simulink model "my_DC_motor_model"  (R2022b)
settings: Solver=FixedStepAuto  StartTime=0.0  StopTime=5  FixedStep=0.0001  RelTol=1e-3
values from neighbouring files (symbols this model uses):
  B_motor = 1.9099e-4    (= 0.00019099)    [DC_motor_init.m]    (also in LOAD_ROBOT_DATA.m = 0.000678; circular_interp.m = 0.000678; computed_torque_control.m; create_model_tree.m)
  J_rotor = 2118.45e-7    (= 0.000211845)    [DC_motor_init.m]    (also in LOAD_ROBOT_DATA.m = 0.0125; circular_interp.m = 0.0125; computed_torque_control.m; create_model_tree.m)
  Ke = 0.08    [DC_motor_init.m]    (also in LOAD_ROBOT_DATA.m = 0.957; circular_interp.m = 0.957; computed_torque_control.m; create_model_tree.m)
  Kt = 0.08    [DC_motor_init.m]    (also in LOAD_ROBOT_DATA.m = 0.957; circular_interp.m = 0.957; computed_torque_control.m; create_model_tree.m)
  L = 0.90e-3    (= 0.0009)    [DC_motor_init.m]    (also in LOAD_ROBOT_DATA.m = 0.0054; circular_interp.m = 0.0054; computed_torque_control.m; create_model_tree.m)
  R = 0.43    [DC_motor_init.m]    (also in LOAD_ROBOT_DATA.m = 1.45; circular_interp.m = 1.45; computed_torque_control.m; create_model_tree.m)
settings Model: Creator=doann  LastModifiedBy=doann

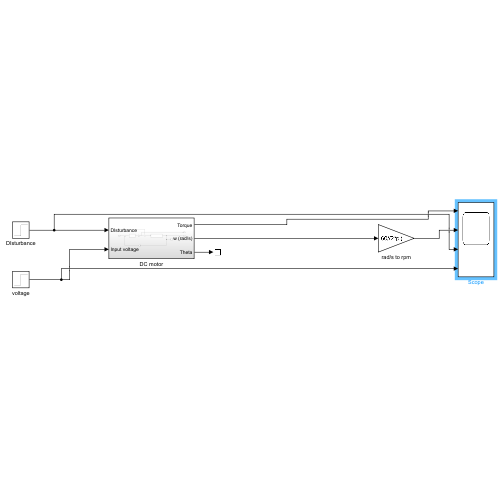
[thumbnail: Simulink's stored preview of the top-level diagram]
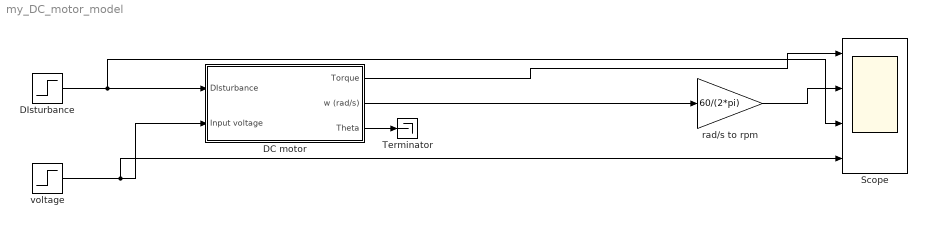
== system my_DC_motor_model ==
  DC motor : Subsystem
  DIsturbance : Step  Time=2.5  After=5  SampleTime=0
  Scope : Scope  NumInputPorts=4
  Terminator : Terminator
  rad/s to rpm : Gain  Gain=60/(2*pi)
  voltage : Step  Time=2  After=12  SampleTime=0
  wires:
  rad/s to rpm/1 -> Scope/2
  DIsturbance/1 -> Scope/3, DC motor/1(DIsturbance)
  voltage/1 -> Scope/4, DC motor/2(Input voltage)
  DC motor/1(Torque) -> Scope/1
  DC motor/2(w (rad/s)) -> rad/s to rpm/1
  DC motor/3(Theta) -> Terminator/1

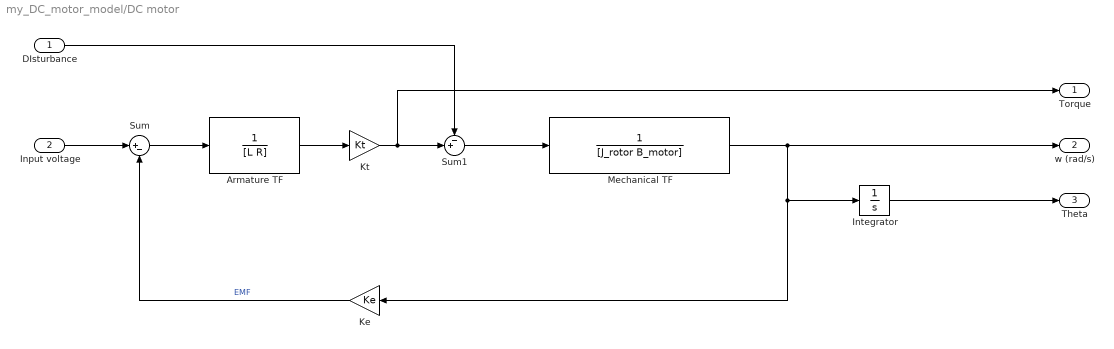
== system my_DC_motor_model/DC motor ==
  DIsturbance : Inport
  Input voltage : Inport  Port=2
  Armature TF : TransferFcn  Denominator=[L R]
  Integrator : Integrator
  Ke : Gain  Gain=Ke
  Kt : Gain  Gain=Kt
  Mechanical TF : TransferFcn  Denominator=[J_rotor B_motor]
  Sum : Sum  Inputs=|+-
  Sum1 : Sum  Inputs=-+|
  Torque : Outport
  w (rad/s) : Outport  Port=2
  Theta : Outport  Port=3
  wires:
  Ke/1 -> Sum/2  "EMF"
  Mechanical TF/1 -> w (rad/s)/1, Ke/1, Integrator/1
  Kt/1 -> Torque/1, Sum1/2
  Sum/1 -> Armature TF/1
  Sum1/1 -> Mechanical TF/1
  Armature TF/1 -> Kt/1
  DIsturbance/1 -> Sum1/1
  Integrator/1 -> Theta/1
  Input voltage/1 -> Sum/1
